simulink model "elevator_work1"  (R2014a)
settings: Solver=ode45  StartTime=0.0  StopTime=10000000  RelTol=1e-3
libraries: simulink x5
settings Model: Creator=Rishabh  LastModifiedBy=Rishabh

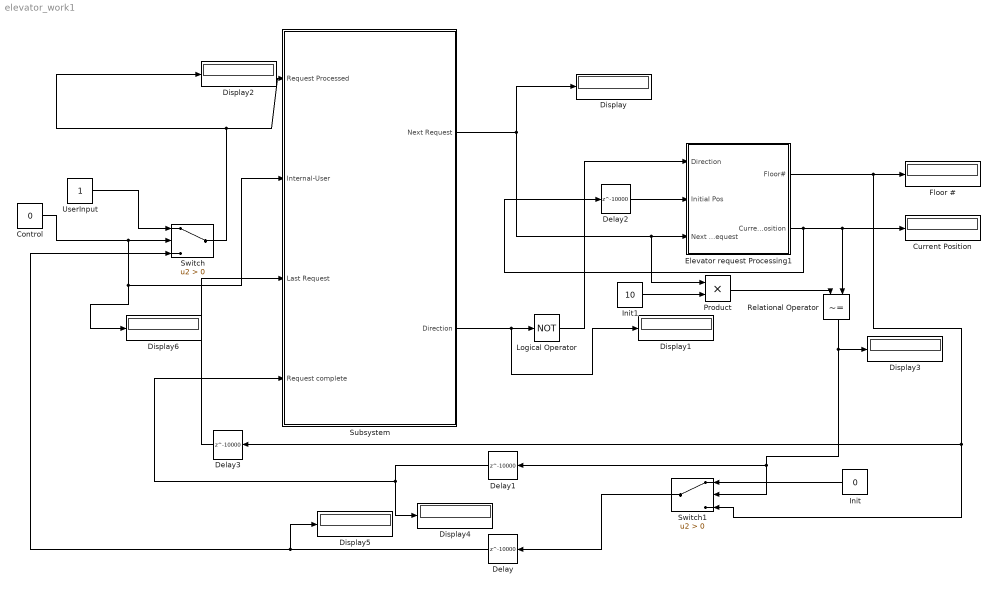
== system elevator_work1 ==
  Control : Constant  Value=0
  Current Position : Display
  Delay{,1..3} (4 alike) : Delay  DelayLength=10000  InitialCondition=0  SampleTime=.00001
  Display{,1..6} (7 alike) : Display
  Elevator request Processing1 : Subsystem
  Floor # : Display
  Init : Constant  Value=0
  Init1 : Constant  Value=10
  Logical Operator : Logic  Operator=NOT  AllPortsSameDT=off  OutDataTypeStr=boolean
  Product : Product
  Relational Operator : RelationalOperator  Operator=~=  OutDataTypeStr=boolean
  Subsystem : Subsystem
  Switch : Switch  Criteria=u2 > Threshold
  Switch1 : Switch  Criteria=u2 > Threshold
  UserInput : Constant
  wires:
  Subsystem/2(Direction) -> Display1/1, Logical Operator/1
  Subsystem/1(Next Request) -> Display/1, Product/1, Elevator request Processing1/3(Next Request)
  Switch1/1 -> Delay/1
  Switch/1 -> Subsystem/1(Request Processed), Display2/1
  Elevator request Processing1/1(Floor#) -> Delay3/1, Switch1/3, Floor #/1
  UserInput/1 -> Switch/1
  Relational Operator/1 -> Switch1/2, Delay1/1, Display3/1
  Init/1 -> Switch1/1
  Delay/1 -> Display5/1, Switch/3
  Delay1/1 -> Display4/1, Subsystem/4(" Request complete")
  Delay2/1 -> Elevator request Processing1/2(Initial Pos)
  Logical Operator/1 -> Elevator request Processing1/1(Direction)
  Elevator request Processing1/2(Current Position) -> Delay2/1, Current Position/1, Relational Operator/2
  Init1/1 -> Product/2
  Product/1 -> Relational Operator/1
  Control/1 -> Display6/1, Subsystem/2(Internal-User), Switch/2
  Delay3/1 -> Subsystem/3(Last Request)

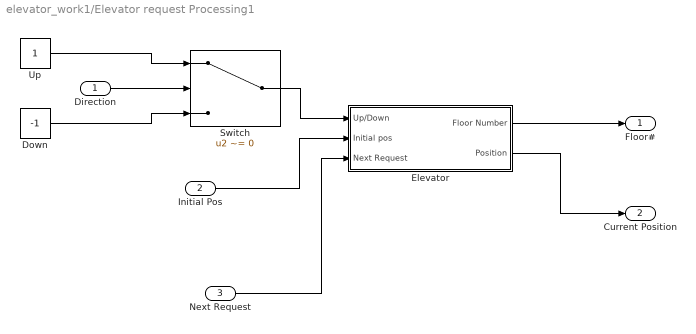
== system elevator_work1/Elevator request Processing1 ==
  Direction : Inport
  Initial Pos : Inport  Port=2
  Next Request : Inport  Port=3
  Down : Constant  Value=-1
  Elevator : Subsystem
  Switch : Switch  Criteria=u2 ~= 0
  Up : Constant
  Floor# : Outport
  Current Position : Outport  Port=2
  wires:
  Up/1 -> Switch/1
  Direction/1 -> Switch/2
  Switch/1 -> Elevator/1(Up/Down)
  Down/1 -> Switch/3
  Next Request/1 -> Elevator/3(Next Request)
  Elevator/1(Floor Number) -> Floor#/1
  Elevator/2(Position) -> Current Position/1
  Initial Pos/1 -> Elevator/2(Initial pos)

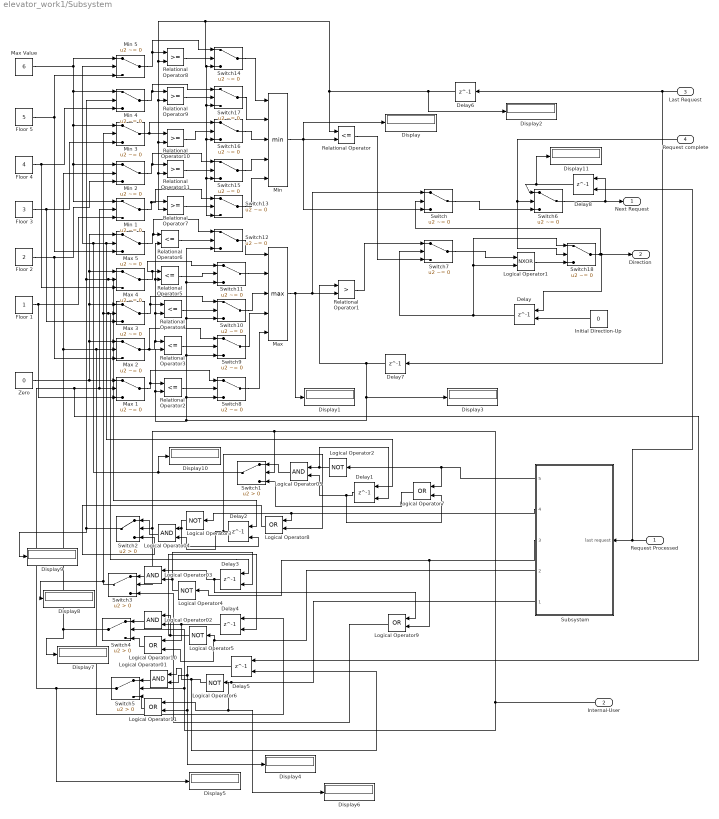
== system elevator_work1/Subsystem ==
  Request Processed : Inport
  Internal-User : Inport  Port=2
  Last Request : Inport  Port=3
  " Request complete" : Inport  Port=4
  Delay : Delay  DelayLength=1  InitialConditionSource=Input port  InitialCondition=0  SampleTime=1
      settings: InputPortMap=u0,p4
  Delay{1..5} (5 alike) : Delay  DelayLength=1  InitialConditionSource=Input port  InitialCondition=1  SampleTime=.1
      settings: InputPortMap=u0,p4
  Delay6 : Delay  DelayLength=1  InitialCondition=0
  Delay7 : Delay  DelayLength=1  InitialCondition=0
  Delay8 : Delay  DelayLength=1  InitialConditionSource=Input port  InitialCondition=0  SampleTime=.1
      settings: InputPortMap=u0,p4
  Display{,1..11} (12 alike) : Display
  Floor 1 : Constant
  Floor 2 : Constant  Value=2
  Floor 3 : Constant  Value=3
  Floor 4 : Constant  Value=4
  Floor 5 : Constant  Value=5
  Initial Direction-Up : Constant  Value=0  OutDataTypeStr=boolean
  Logical Operato04 : Logic  AllPortsSameDT=off  OutDataTypeStr=boolean
  Logical Operator01 : Logic  AllPortsSameDT=off  OutDataTypeStr=boolean
  Logical Operator02 : Logic  AllPortsSameDT=off  OutDataTypeStr=boolean
  Logical Operator03 : Logic  AllPortsSameDT=off  OutDataTypeStr=boolean
  Logical Operator05 : Logic  AllPortsSameDT=off  OutDataTypeStr=boolean
  Logical Operator1 : Logic  Operator=NXOR  AllPortsSameDT=off  OutDataTypeStr=boolean
  Logical Operator{7..11} (5 alike) : Logic  Operator=OR  AllPortsSameDT=off  OutDataTypeStr=boolean
  Logical Operator{2..6} (5 alike) : Logic  Operator=NOT  AllPortsSameDT=off  OutDataTypeStr=boolean
  Max : MinMax  Function=max  Inputs=5
  Max {1..5} (5 alike) : Switch  Criteria=u2 ~= 0
  Max Value : Constant  Value=6
  Min : MinMax  Inputs=5
  Min {1..4} (4 alike) : Switch  Criteria=u2 ~= 0
  Min 5 : Switch  Criteria=u2 ~= 0  Threshold=5
  Relational Operator{,2..6} (6 alike) : RelationalOperator  Operator=<=  OutDataTypeStr=boolean
  Relational Operator1 : RelationalOperator  Operator=>  OutDataTypeStr=boolean
  Relational Operator{7..11} (5 alike) : RelationalOperator  OutDataTypeStr=boolean
  Subsystem : Subsystem
  Switch{,6..18} (14 alike) : Switch  Criteria=u2 ~= 0
  Switch{1..5} (5 alike) : Switch  Criteria=u2 > Threshold
  Zero : Constant  Value=0
  Next Request : Outport
  Direction : Outport  Port=2
  wires:
  Initial Direction-Up/1 -> Delay/2
  Floor 2/1 -> Max 2/3, Min 2/3
  Min 3/1 -> Switch16/1, Relational Operator10/1
  Switch7/1 -> Logical Operator1/1
  Delay/1 -> Switch7/2, Switch18/1, Logical Operator1/2
  Max 4/1 -> Relational Operator5/1, Switch11/1
  Min 1/1 -> Switch13/1, Relational Operator7/1
  Min 2/1 -> Switch15/1, Relational Operator11/1
  Relational Operator1/1 -> Switch7/1
  Floor 1/1 -> Max 1/3, Min 1/3
  Min/1 -> Display/1, Relational Operator/2, Switch/3
  Floor 3/1 -> Max 3/3, Min 3/3
  Max Value/1 -> Min 5/1, Min 4/1, Min 3/1, Min 2/1, Min 1/1
  Floor 5/1 -> Min 5/3, Max 5/3
  Floor 4/1 -> Max 4/3, Min 4/3
  Max 5/1 -> Switch12/1, Relational Operator6/1
  Max 2/1 -> Switch9/1, Relational Operator6/2, Relational Operator5/2, Relational Operator4/2, Relational Operator3/1
  Max 1/1 -> Switch8/1, Relational Operator2/1
  Min 4/1 -> Switch17/1, Relational Operator9/1
  Zero/1 -> Max 5/1, Max 4/1, Max 3/1, Max 2/1, Max 1/1
  Max 3/1 -> Relational Operator4/1, Switch10/1
  Relational Operator/1 -> Switch7/3
  Max/1 -> Display1/1, Switch/1, Relational Operator1/2
  Request Processed/1 -> Delay8/2, Subsystem/1(last request)
  Switch1/1 -> Display10/1, Min 5/2, Delay1/1, Max 5/2
  Switch2/1 -> Min 4/2, Delay2/1, Max 4/2, Display9/1
  Switch3/1 -> Display8/1, Min 3/2, Delay3/1, Max 3/2
  Switch4/1 -> Min 2/2, Max 2/2, Delay4/1, Display7/1
  Delay1/1 -> Logical Operator7/2, Logical Operator05/2
  Delay2/1 -> Logical Operator8/2, Logical Operato04/2
  Subsystem/2(4) -> Logical Operator8/1, Logical Operator3/1
  Subsystem/3(3) -> Logical Operator9/2, Logical Operator4/1
  Delay3/1 -> Logical Operator9/1, Logical Operator03/1
  Subsystem/4(2) -> Logical Operator10/2, Logical Operator5/1
  Delay4/1 -> Logical Operator10/1, Logical Operator02/2
  Delay5/1 -> Display4/1, Logical Operator11/2, Logical Operator01/2
  Subsystem/5(1) -> Logical Operator11/1, Display6/1, Logical Operator6/1
  Subsystem/1(5) -> Logical Operator7/1, Logical Operator2/1
  Logical Operator2/1 -> Delay1/2, Logical Operator05/1
  Logical Operator3/1 -> Delay2/2, Logical Operato04/1
  Logical Operator4/1 -> Delay3/2, Logical Operator03/2
  Logical Operator5/1 -> Delay4/2, Logical Operator02/1
  Logical Operator6/1 -> Delay5/2, Logical Operator01/1
  Logical Operator7/1 -> Switch1/3
  Logical Operator05/1 -> Switch1/1
  Logical Operato04/1 -> Switch2/1
  Logical Operator8/1 -> Switch2/3
  Logical Operator9/1 -> Switch3/3
  Logical Operator03/1 -> Switch3/1
  Logical Operator02/1 -> Switch4/1
  Logical Operator10/1 -> Switch4/3
  Logical Operator01/1 -> Switch5/1
  Logical Operator11/1 -> Switch5/3
  Internal-User/1 -> Switch3/2, Switch2/2, Switch1/2, Switch4/2, Switch5/2
  Delay6/1 -> Display2/1, Switch13/3, Switch15/3, Switch16/3, Switch17/3, Switch14/3, Relational Operator7/2, Relational Operator11/2, Relational Operator10/2, Relational Operator9/2, Relational Operator8/2, Relational Operator/1
  Delay7/1 -> Display3/1, Switch12/3, Switch11/3, Switch10/3, Switch9/3, Switch8/3, Relational Operator2/2, Relational Operator3/2, Relational Operator1/1
  Last Request/1 -> Delay7/1, Delay6/1
  Switch5/1 -> Display5/1, Min 1/2, Max 1/2, Delay5/1
  Switch6/1 -> Delay8/1, Next Request/1
  Delay8/1 -> Display11/1, Switch6/1
  Switch/1 -> Switch6/3
  Relational Operator2/1 -> Switch8/2
  Switch8/1 -> Max/5
  Relational Operator3/1 -> Switch9/2
  Switch9/1 -> Max/4
  Switch10/1 -> Max/3
  Relational Operator4/1 -> Switch10/2
  Relational Operator5/1 -> Switch11/2
  Switch11/1 -> Max/2
  Relational Operator6/1 -> Switch12/2
  Switch12/1 -> Max/1
  Min 5/1 -> Relational Operator8/1, Switch14/1
  Relational Operator8/1 -> Switch14/2
  Switch14/1 -> Min/1
  Switch17/1 -> Min/2
  Switch16/1 -> Min/3
  Switch15/1 -> Min/4
  Switch13/1 -> Min/5
  Relational Operator7/1 -> Switch13/2
  Relational Operator11/1 -> Switch15/2
  Relational Operator10/1 -> Switch16/2
  Relational Operator9/1 -> Switch17/2
  Logical Operator1/1 -> Switch18/3
  Switch18/1 -> Switch/2, Delay/1, Direction/1
  " Request complete"/1 -> Switch18/2, Switch6/2

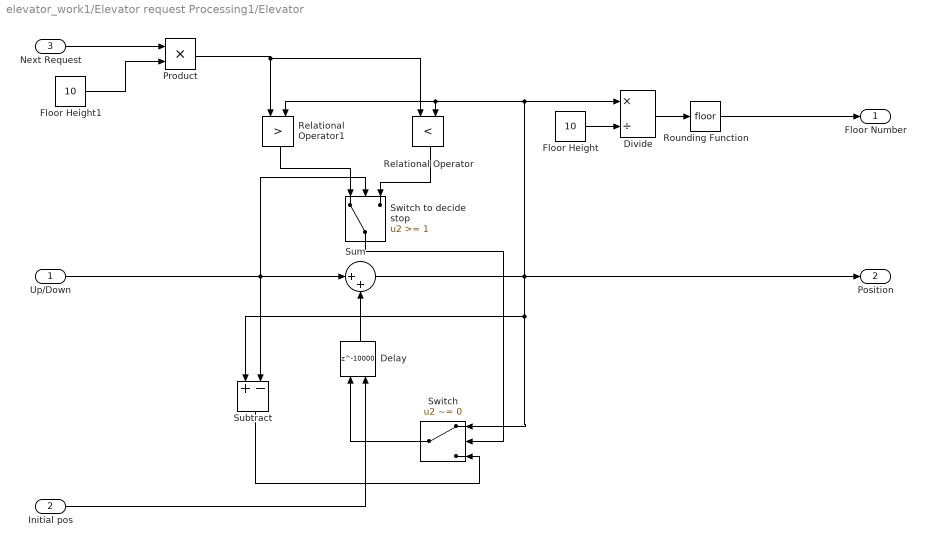
== system elevator_work1/Elevator request Processing1/Elevator ==
  Up/Down : Inport
  Initial pos : Inport  Port=2
  Next Request : Inport  Port=3
  Delay : Delay  DelayLength=10000  InitialConditionSource=Input port  InitialCondition=2  SampleTime=.00001
      settings: InputPortMap=u0,p4
  Divide : Product  Inputs=*/  RndMeth=Nearest  LockScale=on
  Floor Height : Constant  Value=10
  Floor Height1 : Constant  Value=10
  Product : Product
  Relational Operator : RelationalOperator  Operator=<  OutDataTypeStr=boolean
  Relational Operator1 : RelationalOperator  Operator=>  OutDataTypeStr=boolean
  Rounding Function : Rounding
  Subtract : Sum  Inputs=+-
  Sum : Sum  Inputs=|++
  Switch : Switch  Criteria=u2 ~= 0
  Switch to decide stop : Switch  Threshold=1
  Floor Number : Outport
  Position : Outport  Port=2
  wires:
  Delay/1 -> Sum/2
  Up/Down/1 -> Switch to decide stop/2, Sum/1, Subtract/2
  Sum/1 -> Position/1, Subtract/1, Switch/1, Relational Operator1/2, Relational Operator/2, Divide/1
  Divide/1 -> Rounding Function/1
  Floor Height/1 -> Divide/2
  Rounding Function/1 -> Floor Number/1
  Relational Operator/1 -> Switch to decide stop/3
  Switch/1 -> Delay/1
  Relational Operator1/1 -> Switch to decide stop/1
  Switch to decide stop/1 -> Switch/2
  Subtract/1 -> Switch/3
  Initial pos/1 -> Delay/2
  Next Request/1 -> Product/1
  Product/1 -> Relational Operator/1, Relational Operator1/1
  Floor Height1/1 -> Product/2

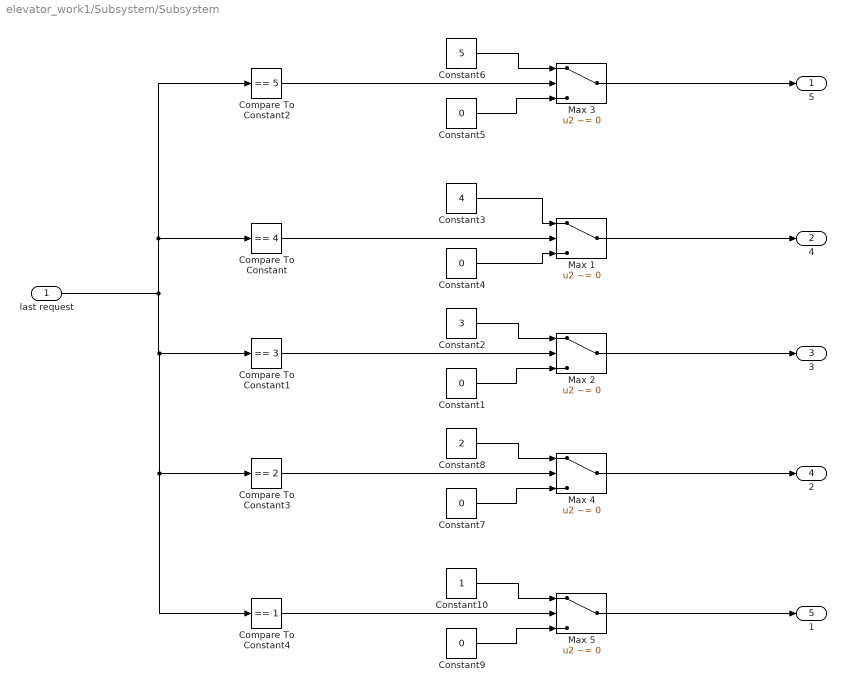
== system elevator_work1/Subsystem/Subsystem ==
  last request : Inport
  Compare To Constant : simulink/Logic and Bit Operations/Compare To Constant  relop===  const=4  OutDataTypeStr=boolean
  Compare To Constant1 : simulink/Logic and Bit Operations/Compare To Constant  relop===  const=3  OutDataTypeStr=boolean
  Compare To Constant2 : simulink/Logic and Bit Operations/Compare To Constant  relop===  const=5  OutDataTypeStr=boolean
  Compare To Constant3 : simulink/Logic and Bit Operations/Compare To Constant  relop===  const=2  OutDataTypeStr=boolean
  Compare To Constant4 : simulink/Logic and Bit Operations/Compare To Constant  relop===  const=1  OutDataTypeStr=boolean
  Constant{1,4..5,7,9} (5 alike) : Constant  Value=0
  Constant10 : Constant
  Constant2 : Constant  Value=3
  Constant3 : Constant  Value=4
  Constant6 : Constant  Value=5
  Constant8 : Constant  Value=2
  Max {1..5} (5 alike) : Switch  Criteria=u2 ~= 0
  5 : Outport
  4 : Outport  Port=2
  3 : Outport  Port=3
  2 : Outport  Port=4
  1 : Outport  Port=5
  wires:
  Max 3/1 -> 5/1
  Constant5/1 -> Max 3/3
  Constant6/1 -> Max 3/1
  Compare To Constant2/1 -> Max 3/2
  Compare To Constant4/1 -> Max 5/2
  Max 5/1 -> 1/1
  Constant9/1 -> Max 5/3
  last request/1 -> Compare To Constant2/1, Compare To Constant/1, Compare To Constant4/1, Compare To Constant3/1, Compare To Constant1/1
  Constant10/1 -> Max 5/1
  Constant1/1 -> Max 2/3
  Max 1/1 -> 4/1
  Constant3/1 -> Max 1/1
  Compare To Constant1/1 -> Max 2/2
  Max 4/1 -> 2/1
  Constant7/1 -> Max 4/3
  Constant8/1 -> Max 4/1
  Compare To Constant3/1 -> Max 4/2
  Constant2/1 -> Max 2/1
  Compare To Constant/1 -> Max 1/2
  Max 2/1 -> 3/1
  Constant4/1 -> Max 1/3
